simulink model "Hydraulic_Lift"  (R2013a)
settings: Solver=ode23t  StartTime=0.0  StopTime=20  MaxStep=0.02  RelTol=1e-3  AbsTol=1e-4
PreLoadFcn:
  | %cylinder_length = 15*2;
  | %piston_length = 15*2;
  | %leg_length = 15*2;
  | %platform_length = 25*2;
PostLoadFcn:
  | warning off sm:compiler:topologyAnalysis:DanglingBlock
  | warning off Simulink:SL_SolverMaskedZC;
  | warning off Simulink:SL_SolverIgnoredZCBracketing;
  | warning off Simulink:Engine:SolverMinStepNonlinearIterWarnForDAE;
  | warning off simscape:compiler:sli:init:SolverNotRecommended
  | warning off Simulink:Engine:UsingDiscreteSolver
  | load_system('Cylinder_Lib');
  | load_system('Motor_Lib');
  | load_system('Valve_Lib');
  | load_system('Load_Lib');
undefined symbols (not defined in the file or in its folder): Local, Scissor_Lift_Param, sigbuilder_block, X, Y, Z
libraries: fl_lib x80, sm_lib x41, Scissor_Parts_Lib x24, nesl_utility x8, Custom_lib x1
(part 1 of 2)
Description:
  | Copyright 2013 The MathWorks, Inc.
settings Model: Creator=smiller  LastModifiedBy=smiller
settings OptimizationCC: ExpressionDepthLimit=2147483647
settings SimscapeCC: SimscapeLogType=all  SimscapeLogSimulationStatistics=on  SimscapeLogLimitData=off
settings ExplorerConfigSet: InternalSimMechanicsExplorerSettings="<ExplorerConfiguration><canonicalview>default</canonicalview><TilePanel><TileInfo><Tiles Columns=\"1\" Count=\"1\" Rows=\"1\"><Column Left=\"2\" Weight=\"1\"/><Column Left=\"424\"/><Row Top=\"2\" Weight=\"1\"/><Row Top=\"524\"/><Tile Height=\"1\" Width=\"1\" X=\"0\" Y=\"0\"/></Tiles></TileInfo><SceneInfo><SceneViewer><BGColor><R>0.94901961088180542</R><G>0.94901961088180542</G><B>0.94901961088180542</B></BGColor><Camera><Position><X>2.491802304979692</X><Y>-4.0942122250600148</Y><Z>2.1539121347282051</Z></Position><Center><X>-0.87035068779914659</X><Y>-0.07952129192366976</Y><Z>1.2617431921759128</Z></Center><Up><X>-0.14501327569823058</X><Y>0.097366663542222315</Y><Z>0.98462728110789444</Z></Up><Left>-1.3650000751018525</Left><Right>1.3650000751018525</Right><Bottom>-1.2464621901512147</Bottom><Top>1.2464621901512147</Top></Camera></SceneViewer></SceneInfo></TilePanel></ExplorerConfiguration>"

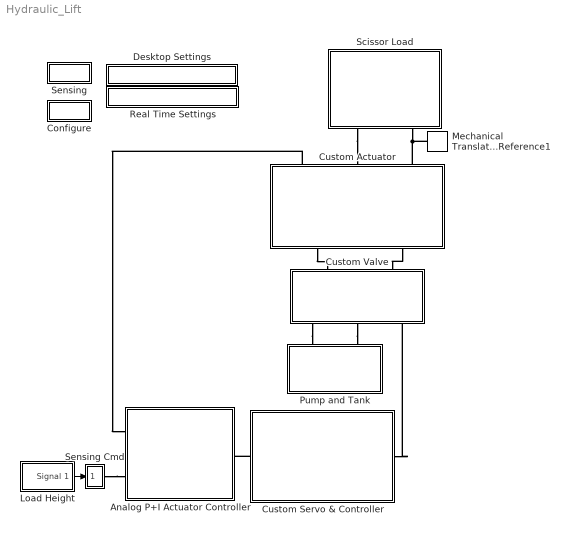
== system Hydraulic_Lift ==
  Analog P+I Actuator Controller : Subsystem
      mask Display: image(imread('Analog_PI_Controller_IMAGE.jpg'))
  Configure : Subsystem
      settings: OpenFcn=|
      | set_param([bdroot '/Configure/Commands'],'Location',[543 426 1032 720]);
      | open_system([bdroot '/Configure/Commands'],'window');
  Custom Actuator : Subsystem  mask(Double-Acting Hydraulic Actuator){A=5e-4, V=10e-6, PA=200, PB=0, T=200}
      mask prompts: A "Piston area (m^2)"; V "Chamber dead volume (m^3)"; PA "Positive-acting chamber A inital pressure (bar)"; PB "Negative-acting chamber B inital pressure (bar)"; T "Piston Travel (mm)"
      mask help: Models a double-acting hydraulic actuator using foundation libary blocks
      mask Display: image(imread('Double_Acting_Cylinder_Custom_IMAGE.jpg'));
  Custom Servo & Controller : Subsystem  mask{G=0.5e-3/(pi/2), J=1e-4, lambda=0.01, R=10, L=2.5, Kt=0.04, R_controller=[10e3 10e3 10e3 100e3 50 100e3 10e3], x_max=0.5}
      mask prompts: G "Spool displacement per motor rotation"; J "Total inertia reflected to motor (kg m^2)"; lambda "Total damping reflected to motor (Nm/(rad/s))"; R "Torque motor winding resistance (ohms)"; L "Torque motor winding inductance (H)"; Kt "Torque motor torque constant (Nm/A)"; R_controller "Motor controller resistance values [R1 R2 R3 R4 R5 R6 R7] (ohms)"; x_max "Spool displacement limit (mm)"
      mask Display: image(imread('DC_Motor_Custom_IMAGE.jpg'))
  Custom Valve : Subsystem  mask(Single-Stage Servo Valve){K_V=0.5, x_max=0.5, A_max=9, x_lap=0.02, A_leak=0.25}
      mask prompts: K_V "Flow Coefficient:"; x_max "Spool displacement limit (mm)"; A_max "Maximum oriface area (mm^2)"; x_lap "Spool displacement range for leakage (mm)"; A_leak "Leakage area at x=0 (mm^2)"
      mask help: Models a spool valve actuated directly by a torque motor.
      mask Display: image(imread('Four_Way_Valve_Custom_IMAGE.jpg'))
  Desktop Settings : Subsystem
      settings: OpenFcn=|
      | set_param(bdroot,'Solver','ODE23t','MaxStep','0.02');
      | 
      | 
      | tvar_solverBlock = find_system(bdroot, 'SubClassName', 'solver');
      | 
      | for i=1:size(tvar_solverBlock,1)
      | 
      | set_param(char(tvar_solverBlock(i)), 'UseLocalSolver','off','DoFixedCost','off');
      | end
      | 
      | clear tvar_solverBlock
      mask Display: disp('Desktop Settings')
  Load Height : Subsystem  Tag=STV Subsys  LoadFcn=sigbuilder_block('load');  StartFcn=sigbuilder_block('start');  StopFcn=sigbuilder_block('stop');  ClipboardFcn=sigbuilder_block('clipboard');  mask(Sigbuilder block){}
      mask help: Sigbuilder GUI
      mask init:
      | if ~strcmp(get_param(bdroot(gcbh),'SimulationStatus'),'stopped') tuvar = sigbuilder_block('maskInit'); end
      settings: CopyFcn=sigbuilder_block('copy');  DeleteFcn=sigbuilder_block('delete');  ModelCloseFcn=sigbuilder_block('modelClose');  PreSaveFcn=sigbuilder_block('preSave');  PauseFcn=sigbuilder_block('pause')  ContinueFcn=sigbuilder_block('continue')  NameChangeFcn=sigbuilder_block('namechange');  OpenFcn=sigbuilder_block('open',[181.241 5.58621 330.828 249.517 ]);  CloseFcn=sigbuilder_block('close');
      mask Display: plot(0,0,100,100,[10,10,40,40,10],[80,20,20,80,80],[40,10],[50,50], [40,27,10],[65,72,56],[40,25,25,10],[28,28,43,43]);
  Mechanical Translational Reference1 : fl_lib/Mechanical/Translational Elements/Mechanical Translational Reference  f_Log=off  LocalVarNames=|f  LocalVarDescs=|f  LocalVarLogging=[]
  Pump and Tank : Subsystem
      mask Display: image(imread('Pump_IMAGE.JPG'));
  Real Time Settings : Subsystem
      settings: OpenFcn=|
      | tvar_Nonlinear_Iterations = '4';
      | tvar_StepSize = '0.002';
      | %tvar_LocalSolver = 'NE_TRAPEZOIDAL_ADVANCER';
      | tvar_LocalSolver = 'NE_BACKWARD_EULER_ADVANCER';
      | 
      | set_param(bdroot,'Solver','ode1','FixedStep','auto');
      | 
      | tvar_solverBlock = find_system(bdroot, 'SubClassName', 'solver');
      | for i=1:size(tvar_solverBlock,1)
      | 
      | set_param(char(tvar_solverBlock(i)), 'UseLocalSolver','on','DoFixedCost','on','MaxNonlinIter',tvar_Nonlinear_Iterations,'LocalSolverChoice',tvar_LocalSolver,'LocalSolverSampleTime',tvar_StepSize);
      | end
      | clear tvar_Nonlinear_Iterations tvar_StepSize tvar_LocalSolver tvar_solverBlock
      mask Display: disp('Real Time Settings')
  Scissor Load : Subsystem
      mask Display: image(imread('Load_Scissor_IMAGE.JPG'));
  Sensing : Subsystem
  Sensing Cmd : Subsystem
      mask Display: disp('S')
  wires:
  Load Height/1(Signal 1) -> Sensing Cmd/1(In1)
  connections:
  Mechanical Translational Reference1/LConn1 -- Scissor Load/LConn2 -- Custom Actuator/RConn3
  Custom Actuator/LConn1 -- Custom Valve/RConn1
  Custom Servo & Controller/LConn1 -- Analog P+I Actuator Controller/RConn1
  Custom Actuator/LConn2 -- Custom Valve/RConn2
  Custom Actuator/RConn1 -- Analog P+I Actuator Controller/LConn1
  Sensing Cmd/RConn1 -- Analog P+I Actuator Controller/LConn2
  Scissor Load/LConn1 -- Custom Actuator/RConn2
  Custom Valve/LConn1 -- Pump and Tank/RConn1
  Custom Valve/LConn2 -- Pump and Tank/RConn2
  Custom Servo & Controller/RConn1 -- Custom Valve/LConn3

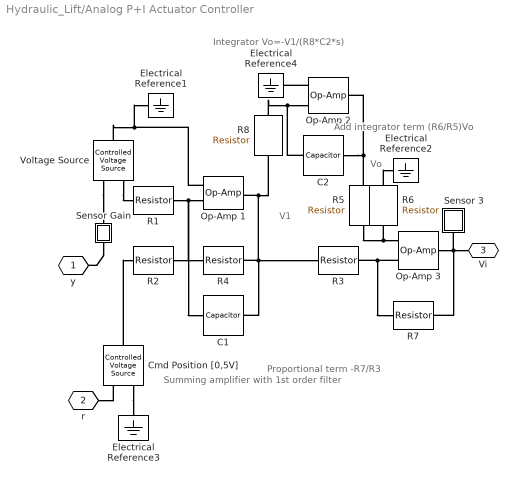
== system Hydraulic_Lift/Analog P+I Actuator Controller ==
  note: Summing amplifier
      | with 1st order filter
  note: Integrator
      | Vo=-V1/(R8*C2*s)
  note: Proportional
      | term -R7/R3
  note: Add integrator
      | term (R6/R5)Vo
  note: Vo
  note: V1
  C1 : fl_lib/Electrical/Electrical Elements/Capacitor  c=0.15e-06 F  v0=0 V  r=1e-06 Ohm  g=0 1/Ohm  i_Log=off  v_Log=off  vc_Log=off  LocalVarNames=|current|voltage|power  LocalVarDescs=|Capacitor current (A)|Voltage across capacitor (V)|Power (W)  LocalVarLogging=[0 0 0]
  C2 : fl_lib/Electrical/Electrical Elements/Capacitor  c=100e-06 F  v0=0 V  r=1e-06 Ohm  g=0 1/Ohm  i_Log=off  v_Log=off  vc_Log=off  LocalVarNames=|current|voltage|power  LocalVarDescs=|Capacitor current (A)|Voltage across capacitor (V)|Power (W)  LocalVarLogging=[0 0 0]
  Cmd Position [0,5V] : fl_lib/Electrical/Electrical Sources/Controlled Voltage Source  i_Log=off  v_Log=off  LocalVarNames=|current|voltage|power  LocalVarDescs=|Current (A)|Voltage (V)|Power (W)  LocalVarLogging=[0 0 0]
  Electrical Reference{1..4} (4 alike) : fl_lib/Electrical/Electrical Elements/Electrical Reference  i_Log=off  LocalVarNames=|i  LocalVarDescs=|i  LocalVarLogging=[]
  Op-Amp 1 : fl_lib/Electrical/Electrical Elements/Op-Amp  i1_Log=off  v1_Log=off  outI_Log=off  LocalVarNames=|i1|v1|outI  LocalVarDescs=|i1|v1|outI  LocalVarLogging=[]
  Op-Amp 2 : fl_lib/Electrical/Electrical Elements/Op-Amp  i1_Log=off  v1_Log=off  outI_Log=off  LocalVarNames=|i1|v1|outI  LocalVarDescs=|i1|v1|outI  LocalVarLogging=[]
  Op-Amp 3 : fl_lib/Electrical/Electrical Elements/Op-Amp  i1_Log=off  v1_Log=off  outI_Log=off  LocalVarNames=|i1|v1|outI  LocalVarDescs=|i1|v1|outI  LocalVarLogging=[]
  R{1..3,5..6,8} (6 alike) : fl_lib/Electrical/Electrical Elements/Resistor  R=10e3 Ohm  i_Log=off  v_Log=off  LocalVarNames=|current|voltage|power  LocalVarDescs=|Resistor current (A)|Voltage across resistor (V)|Power (W)  LocalVarLogging=[0 0 0]
  R4 : fl_lib/Electrical/Electrical Elements/Resistor  R=5.7e3 Ohm  i_Log=off  v_Log=off  LocalVarNames=|current|voltage|power  LocalVarDescs=|Resistor current (A)|Voltage across resistor (V)|Power (W)  LocalVarLogging=[0 0 0]
  R7 : fl_lib/Electrical/Electrical Elements/Resistor  R=20e3 Ohm  i_Log=off  v_Log=off  LocalVarNames=|current|voltage|power  LocalVarDescs=|Resistor current (A)|Voltage across resistor (V)|Power (W)  LocalVarLogging=[0 0 0]
  Sensor Gain : Subsystem
      mask Display: disp('G')
  Sensor 3 : Subsystem
      mask Display: disp('S')
  Voltage Source : fl_lib/Electrical/Electrical Sources/Controlled Voltage Source  i_Log=off  v_Log=off  LocalVarNames=|current|voltage|power  LocalVarDescs=|Current (A)|Voltage (V)|Power (W)  LocalVarLogging=[0 0 0]
  y : PMIOPort  Tag=PMCPort  Port=1  Side=Left
  r : PMIOPort  Tag=PMCPort  Port=2  Side=Left
  Vi : PMIOPort  Port=3  Side=Right
  connections:
  r/RConn1 -- Cmd Position [0,5V]/RConn1
  Vi/RConn1 -- R7/RConn1 -- Op-Amp 3/RConn1 -- Sensor 3/LConn1
  R1/RConn1 -- R2/RConn1 -- R4/LConn1 -- C1/LConn1 -- Op-Amp 1/LConn2
  R4/RConn1 -- R3/LConn1 -- C1/RConn1 -- R8/LConn1 -- Op-Amp 1/RConn1
  R8/RConn1 -- C2/LConn1 -- Op-Amp 2/LConn2
  C2/RConn1 -- R5/LConn1 -- Op-Amp 2/RConn1
  Op-Amp 1/LConn1 -- Voltage Source/LConn1 -- Electrical Reference1/LConn1
  R5/RConn1 -- R6/LConn1 -- Op-Amp 3/LConn1
  Op-Amp 3/LConn2 -- R7/LConn1 -- R3/RConn1
  Voltage Source/RConn2 -- R1/LConn1
  Cmd Position [0,5V]/LConn1 -- R2/LConn1
  Cmd Position [0,5V]/RConn2 -- Electrical Reference3/LConn1
  R6/RConn1 -- Electrical Reference2/LConn1
  Op-Amp 2/LConn1 -- Electrical Reference4/LConn1
  Voltage Source/RConn1 -- Sensor Gain/RConn1
  Sensor Gain/LConn1 -- y/RConn1

== system Hydraulic_Lift/Configure ==
  Commands : Subsystem

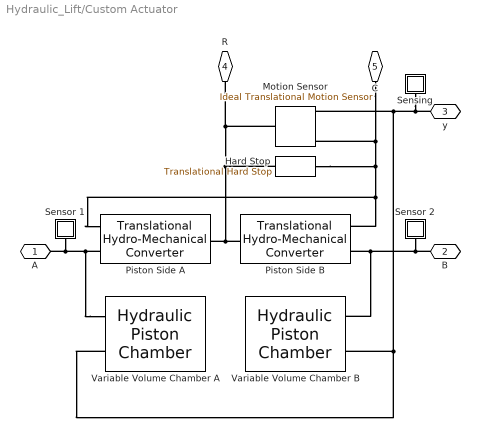
== system Hydraulic_Lift/Custom Actuator ==
  " Motion Sensor" : fl_lib/Mechanical/Mechanical Sensors/Ideal Translational Motion Sensor  offset=Scissor_Lift_Param.Initial_Cyl_Ext mm  v_Log=off  f_Log=off  x_Log=off  LocalVarNames=|v|f|x  LocalVarDescs=|v|f|x  LocalVarLogging=[]
  Hard Stop : fl_lib/Mechanical/Translational Elements/Translational Hard Stop  upper_bnd=T/2 mm  lower_bnd=-T/2 mm  stiff_up=1e7 N/m  stiff_low=1e7 N/m  D_up=1500 N/(m/s)  D_low=1500 N/(m/s)  initial_position=0 m  f_Log=off  v_Log=off  x_Log=off  LocalVarNames=|f|v|x  LocalVarDescs=|f|v|x  LocalVarLogging=[0 0 0]
  Piston Side A : fl_lib/Hydraulic/Hydraulic Elements/Translational Hydro-Mechanical Converter  area=A m^2  or=1  dir=1  f_Log=off  q_Log=off  LocalVarNames=|flow_rate|pressure|force|power  LocalVarDescs=|Flow rate into the chamber (m^3/s)|Pressure at the inlet (Pa)|Output force (N)|Power (W)  LocalVarLogging=[0 0 0 0]
  Piston Side B : fl_lib/Hydraulic/Hydraulic Elements/Translational Hydro-Mechanical Converter  area=A m^2  or=2  dir=1  f_Log=off  q_Log=off  LocalVarNames=|flow_rate|pressure|force|power  LocalVarDescs=|Flow rate into the chamber (m^3/s)|Pressure at the inlet (Pa)|Output force (N)|Power (W)  LocalVarLogging=[0 0 0 0]
  Sensing : Subsystem
      mask Display: disp('S')
  Sensor 1 : Subsystem
      mask Display: disp('S')
  Sensor 2 : Subsystem
      mask Display: disp('S')
  Variable Volume Chamber A : fl_lib/Hydraulic/Hydraulic Elements/Hydraulic Piston Chamber  area=A m^2  init_pos=0 m  or=1  V_dead=V m^3  k_sh=1.4  initial_pressure=PA bar  x_or=1  p_a=101325.0 Pa  chamber_flow_rate_Log=off  pressure_chamber_Log=off  LocalVarNames=|flow_rate|pressure|volume|fl_volume  LocalVarDescs=|Flow rate into the chamber (m^3/s)|Pressure at the inlet (Pa)|Instantaneous chamber volume (m^3)|Compressed fluid volume (m^3)  LocalVarLogging=[0 0 0 0]
  Variable Volume Chamber B : fl_lib/Hydraulic/Hydraulic Elements/Hydraulic Piston Chamber  area=A m^2  init_pos=0 m  or=2  V_dead=V m^3  k_sh=1.4  initial_pressure=PB bar  x_or=1  p_a=101325.0 Pa  chamber_flow_rate_Log=off  pressure_chamber_Log=off  LocalVarNames=|flow_rate|pressure|volume|fl_volume  LocalVarDescs=|Flow rate into the chamber (m^3/s)|Pressure at the inlet (Pa)|Instantaneous chamber volume (m^3)|Compressed fluid volume (m^3)  LocalVarLogging=[0 0 0 0]
  A : PMIOPort  Port=1  Side=Left
  B : PMIOPort  Port=2  Side=Left
  y : PMIOPort  Port=3  Side=Right
  R : PMIOPort  Port=4  Side=Right
  C : PMIOPort  Port=5  Side=Right
  connections:
  Variable Volume Chamber A/LConn1 -- Sensing/LConn1 -- y/RConn1 -- " Motion Sensor"/RConn3 -- Variable Volume Chamber B/LConn1
  " Motion Sensor"/LConn1 -- R/RConn1 -- Piston Side A/RConn1 -- Piston Side B/RConn1 -- Hard Stop/LConn1
  Piston Side A/LConn1 -- Hard Stop/RConn1 -- C/RConn1 -- " Motion Sensor"/RConn1 -- Piston Side B/LConn1
  Variable Volume Chamber B/LConn2 -- Sensor 2/LConn1 -- B/RConn1 -- Piston Side B/LConn2
  Variable Volume Chamber A/LConn2 -- Piston Side A/LConn2 -- A/RConn1 -- Sensor 1/LConn1

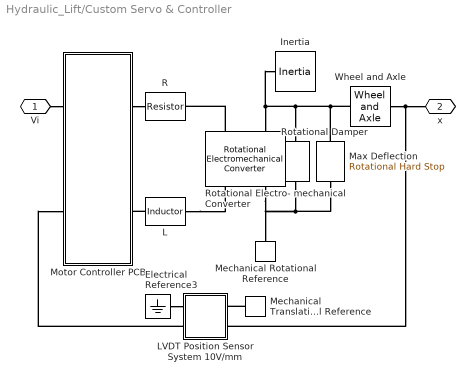
== system Hydraulic_Lift/Custom Servo & Controller ==
  Electrical Reference3 : fl_lib/Electrical/Electrical Elements/Electrical Reference  i_Log=off  LocalVarNames=|i  LocalVarDescs=|i  LocalVarLogging=[]
  Inertia : fl_lib/Mechanical/Rotational Elements/Inertia  inertia=J kg*m^2  initial_velocity=0 rad/s  t_Log=off  LocalVarNames=|torque|velocity  LocalVarDescs=|Inertia torque (N*m)|Inertia absolute velocity (rad/s)  LocalVarLogging=[0 0]
  L : fl_lib/Electrical/Electrical Elements/Inductor  l=L H  i0=0 A  r=0 Ohm  g=1e-09 1/Ohm  i_Log=off  v_Log=off  i_L_Log=off  LocalVarNames=|current|voltage|power  LocalVarDescs=|Inductor current (A) |Voltage across inductor (V)|Power (W)  LocalVarLogging=[0 0 0]
  LVDT Position Sensor System 10V/mm : Subsystem
  Max Deflection : fl_lib/Mechanical/Rotational Elements/Rotational Hard Stop  upper_bnd=x_max*1e-3/G rad  lower_bnd=-x_max*1e-3/G rad  stiff_up=1e+06 N*m/rad  stiff_low=1e+06 N*m/rad  D_up=0.05 N*m/(rad/s)  D_low=0.05 N*m/(rad/s)  initial_angle=0 rad  t_Log=off  w_Log=off  phi_Log=off  LocalVarNames=|contact_torque|rel_angle  LocalVarDescs=|Contact torque (N*m)|Slider-case relative angle (rad)  LocalVarLogging=[0 0]
  Mechanical Rotational Reference : fl_lib/Mechanical/Rotational Elements/Mechanical Rotational Reference  t_Log=off  LocalVarNames=|t  LocalVarDescs=|t  LocalVarLogging=[]
  Mechanical Translational Reference : fl_lib/Mechanical/Translational Elements/Mechanical Translational Reference  f_Log=off  LocalVarNames=|f  LocalVarDescs=|f  LocalVarLogging=0
  Motor Controller PCB : Subsystem
  R : fl_lib/Electrical/Electrical Elements/Resistor  Tag=Factory Generic  R=R Ohm  i_Log=off  v_Log=off  LocalVarNames=|current|voltage|power  LocalVarDescs=|Resistor current (A)|Voltage across resistor (V)|Power (W)  LocalVarLogging=[0 0 0]
  Rotational Damper : fl_lib/Mechanical/Rotational Elements/Rotational Damper  D=lambda N*m/(rad/s)  t_Log=off  w_Log=off  LocalVarNames=|torque|velocity|power  LocalVarDescs=|Damping torque (N*m)|Damper relative velocity (rad/s)|Power dissipated in the damper (W)  LocalVarLogging=[0 0 0]
  Rotational Electro- mechanical Converter : fl_lib/Electrical/Electrical Elements/Rotational Electromechanical Converter  K=Kt V/(rad/s)  i_Log=off  v_Log=off  t_Log=off  w_Log=off  LocalVarNames=|current|voltage|power|torque|speed  LocalVarDescs=|Current (A)|Voltage (V)|Power (W)|Torque (Nm)|Angular speed (rad/s)  LocalVarLogging=[0 0 0 0 0]
  Wheel and Axle : fl_lib/Mechanical/Mechanisms/Wheel and Axle  R=G m  or=1  orient=1  t_Log=off  f_Log=off  LocalVarNames=|t|f  LocalVarDescs=|t|f  LocalVarLogging=[0 0]
  Vi : PMIOPort  Port=1  Side=Left
  x : PMIOPort  Port=2  Side=Right
  connections:
  LVDT Position Sensor System 10V/mm/RConn2 -- Motor Controller PCB/LConn2
  Electrical Reference3/LConn1 -- LVDT Position Sensor System 10V/mm/RConn1
  Vi/RConn1 -- Motor Controller PCB/LConn1
  Motor Controller PCB/RConn1 -- R/LConn1
  Rotational Electro- mechanical Converter/LConn1 -- R/RConn1
  Max Deflection/RConn1 -- Rotational Damper/RConn1 -- Rotational Electro- mechanical Converter/RConn2 -- Mechanical Rotational Reference/LConn1
  Max Deflection/LConn1 -- Inertia/LConn1 -- Rotational Electro- mechanical Converter/LConn2 -- Rotational Damper/LConn1 -- Wheel and Axle/LConn1
  L/LConn1 -- Motor Controller PCB/RConn2
  L/RConn1 -- Rotational Electro- mechanical Converter/RConn1
  Wheel and Axle/RConn1 -- LVDT Position Sensor System 10V/mm/LConn2 -- x/RConn1
  Mechanical Translational Reference/LConn1 -- LVDT Position Sensor System 10V/mm/LConn1

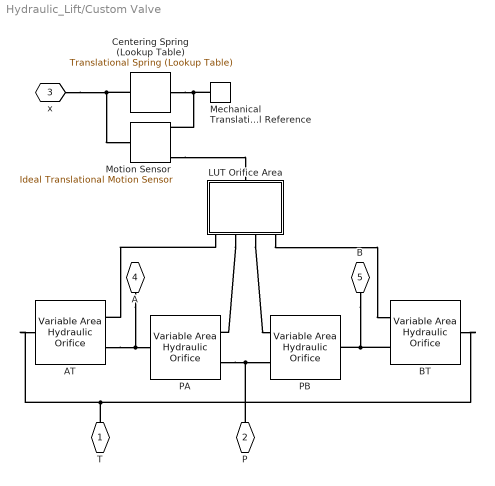
== system Hydraulic_Lift/Custom Valve ==
  AT : fl_lib/Hydraulic/Hydraulic Elements/Variable Area Hydraulic Orifice  C_d=K_V  Re_cr=12  C_d_lam=0.0408  min_area=1e-12 m^2  q_Log=off  p_Log=off  LocalVarNames=|flow_rate|pr_drop|power  LocalVarDescs=|Flow rate through the orifice (m^3)|Pressure drop across the orifice (Pa)|Power dissipated in the orifice (W)  LocalVarLogging=[0 0 0]
  BT : fl_lib/Hydraulic/Hydraulic Elements/Variable Area Hydraulic Orifice  C_d=K_V  Re_cr=12  C_d_lam=0.0408  min_area=1e-12 m^2  q_Log=off  p_Log=off  LocalVarNames=|flow_rate|pr_drop|power  LocalVarDescs=|Flow rate through the orifice (m^3)|Pressure drop across the orifice (Pa)|Power dissipated in the orifice (W)  LocalVarLogging=[0 0 0]
  Centering Spring (Lookup Table) : Custom_lib/Mechanical/Translational Spring (Lookup Table)  xd=[-1 -0.9 0,0.9 1]*x_max mm  kd=[100,10,10,10,100] N/m  x0=0 m  f_Log=off  x_Log=off  v_Log=off  k_Log=off  LocalVarNames=|f|x|v|k  LocalVarDescs=|Force through variable|Displacement|Velocity across variable|Spring Stiffness  LocalVarLogging=[0 0 0 0]
  LUT Orifice Area : Subsystem
  Mechanical Translational Reference : fl_lib/Mechanical/Translational Elements/Mechanical Translational Reference  f_Log=off  LocalVarNames=|f  LocalVarDescs=|f  LocalVarLogging=0
  Motion Sensor : fl_lib/Mechanical/Mechanical Sensors/Ideal Translational Motion Sensor  offset=0 m  v_Log=off  f_Log=off  x_Log=off  LocalVarNames=|v|f|x  LocalVarDescs=|v|f|x  LocalVarLogging=[0 0 0]
  PA : fl_lib/Hydraulic/Hydraulic Elements/Variable Area Hydraulic Orifice  C_d=K_V  Re_cr=12  C_d_lam=0.0408  min_area=1e-12 m^2  q_Log=off  p_Log=off  LocalVarNames=|flow_rate|pr_drop|power  LocalVarDescs=|Flow rate through the orifice (m^3)|Pressure drop across the orifice (Pa)|Power dissipated in the orifice (W)  LocalVarLogging=[0 0 0]
  PB : fl_lib/Hydraulic/Hydraulic Elements/Variable Area Hydraulic Orifice  C_d=K_V  Re_cr=12  C_d_lam=0.0408  min_area=1e-12 m^2  q_Log=off  p_Log=off  LocalVarNames=|flow_rate|pr_drop|power  LocalVarDescs=|Flow rate through the orifice (m^3)|Pressure drop across the orifice (Pa)|Power dissipated in the orifice (W)  LocalVarLogging=[0 0 0]
  T : PMIOPort  Tag=PMCPort  Port=1  Side=Left
  P : PMIOPort  Tag=PMCPort  Port=2  Side=Left
  x : PMIOPort  Tag=PMCPort  Port=3  Side=Left
  A : PMIOPort  Tag=PMCPort  Port=4  Side=Right
  B : PMIOPort  Tag=PMCPort  Port=5  Side=Right
  connections:
  AT/RConn1 -- BT/RConn1 -- T/RConn1
  AT/LConn2 -- PA/RConn1 -- A/RConn1
  PA/LConn2 -- P/RConn1 -- PB/LConn2
  B/RConn1 -- BT/LConn2 -- PB/RConn1
  Mechanical Translational Reference/LConn1 -- Centering Spring (Lookup Table)/RConn1 -- Motion Sensor/RConn1
  LUT Orifice Area/RConn1 -- AT/LConn1
  LUT Orifice Area/RConn4 -- BT/LConn1
  LUT Orifice Area/RConn2 -- PA/LConn1
  LUT Orifice Area/RConn3 -- PB/LConn1
  x/RConn1 -- Centering Spring (Lookup Table)/LConn1 -- Motion Sensor/LConn1
  Motion Sensor/RConn3 -- LUT Orifice Area/LConn1

== system Hydraulic_Lift/Desktop Settings ==

== system Hydraulic_Lift/Load Height ==
  Demux : Demux  Tag=STV Demux  Outputs=1
  FromWs : FromWorkspace  Tag=STV FromWs  VariableName=tuvar  SampleTime=0
      SigBuilderData=|
      | common.afterFinalStr = 'Extrapolate'
      | common.sampleTime = 0
      | dataSet.timeRange = [0 20]
      | dataSet.name = 'Group 1'
      | sbobj.Groups.Name = 'Group 1'
      | sbobj.Groups.Signals.Name = 'Signal 1'
      | sbobj.Groups.Signals.XData = [0 1 3 4 10 12 15 20]
      | sbobj.Groups.Signals.YData = [2.5 2.5 5 5 0 0 2.5 2.5]
      | sbobj.Groups.TimeRange = [0 20]
  Signal 1 : Outport  Tag=STV Outport
  wires:
  Demux/1 -> Signal 1/1
  FromWs/1 -> Demux/1

== system Hydraulic_Lift/Pump and Tank ==
  Custom Hydraulic Fluid : fl_lib/Hydraulic/Hydraulic Utilities/Custom Hydraulic Fluid  density=850 kg/m^3  viscosity_kin=1.8e-05 m^2/s  bulk=8e+08 Pa  alpha=0.005  LocalVarLogging=[]
  Hydraulic Reference : fl_lib/Hydraulic/Hydraulic Elements/Hydraulic Reference  q_Log=off  LocalVarNames=|q  LocalVarDescs=|q  LocalVarLogging=[]
  Pump : fl_lib/Hydraulic/Hydraulic Sources/Hydraulic Pressure Source  q_Log=off  p_Log=off  LocalVarNames=|flow_rate|pr_differential|power  LocalVarDescs=|Flow rate through the source (m^3/s)|Pressure differential across the source (Pa)|Source power (W)  LocalVarLogging=[0 0 0]
  Solver Configuration : nesl_utility/Solver Configuration  PhysicalDomain=network_engine_domain  SubClassName=solver  LeftPortType=input  RightPortType=generic  Accelerate=off  Tones=[]  Harmonics=[]  SimulateNoise=off  Profile=off  UseLocalSampling=off  EnableSwitchedLinearOptims=on  FrequencyDomain=off  UseCCode=off  UseNewInitialization=off  DoDC=off  ResidualTolerance=1e-9  UseLocalSolver=off  LocalSolverChoice=NE_BACKWARD_EULER_ADVANCER  LocalSolverSampleTime=0.002  DoFixedCost=off  MaxNonlinIter=4  MaxModeIter=2  LinearAlgebra=Sparse  DelaysMemoryBudget=1024
  Supply Pressure : Constant  Value=200
  bar : nesl_utility/Simulink-PS Converter  PhysicalDomain=network_engine_domain  SubClassName=ps_input  LeftPortType=input  RightPortType=output  PseudoPeriodic=off  Frequencies=[]  NoiseDistribution=none  NoiseParameters=[]  Unit=bar  AffineConversion=off  InputFiltering=off  SimscapeFilterOrder=1  InputFilterTimeConstant=.001  UdotUserProvided=0
  T : PMIOPort  Port=1  Side=Right
  P : PMIOPort  Port=2  Side=Right
  wires:
  Supply Pressure/1 -> bar/1
  connections:
  bar/RConn1 -- Pump/RConn1
  Pump/RConn2 -- T/RConn1 -- Custom Hydraulic Fluid/RConn1 -- Solver Configuration/RConn1 -- Hydraulic Reference/LConn1
  Pump/LConn1 -- P/RConn1

== system Hydraulic_Lift/Real Time Settings ==

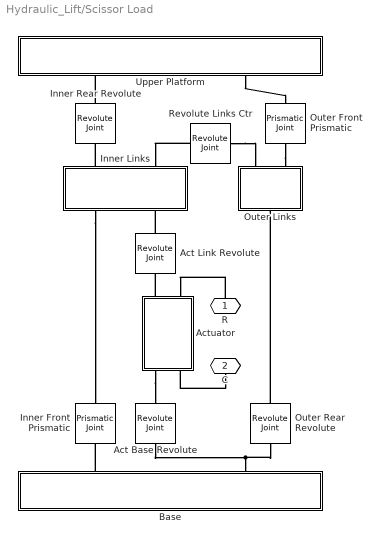
== system Hydraulic_Lift/Scissor Load ==
  Act Base Revolute : sm_lib/Joints/Revolute Joint  SenseConstraintForceX=off  SenseConstraintForceY=off  SenseConstraintForceZ=off  SenseConstraintTorqueX=off  SenseConstraintTorqueY=off  SenseConstraintTorqueZ=off  ConstraintWrenchDir=FollowerOnBase  ConstraintWrenchFrame=BaseFrame  EquilibriumPosition=0  EquilibriumPositionUnits=deg  SpringStiffness=0  SpringStiffnessUnits=N*m/deg  DampingCoefficient=0  DampingCoefficientUnits=N*m/(deg/s)  ActuationMode=NoActuation  SensePosition=off  SenseVelocity=off  SenseAcceleration=off  SenseTorqueForce=off  PositionTargetValue=0  PositionTargetValueUnits=deg  PositionTargetSpecify=off  PositionTargetPriority=High  VelocityTargetValue=0  VelocityTargetValueUnits=deg/s  VelocityTargetSpecify=off  VelocityTargetPriority=High  BlockFunction=simmechanics.library.joints.revolute_joint
  Act Link Revolute : sm_lib/Joints/Revolute Joint  SenseConstraintForceX=off  SenseConstraintForceY=off  SenseConstraintForceZ=off  SenseConstraintTorqueX=off  SenseConstraintTorqueY=off  SenseConstraintTorqueZ=off  ConstraintWrenchDir=FollowerOnBase  ConstraintWrenchFrame=BaseFrame  EquilibriumPosition=0  EquilibriumPositionUnits=deg  SpringStiffness=0  SpringStiffnessUnits=N*m/deg  DampingCoefficient=0  DampingCoefficientUnits=N*m/(deg/s)  ActuationMode=NoActuation  SensePosition=off  SenseVelocity=off  SenseAcceleration=off  SenseTorqueForce=off  PositionTargetValue=0  PositionTargetValueUnits=deg  PositionTargetSpecify=off  PositionTargetPriority=High  VelocityTargetValue=0  VelocityTargetValueUnits=deg/s  VelocityTargetSpecify=off  VelocityTargetPriority=High  BlockFunction=simmechanics.library.joints.revolute_joint
  Actuator : Subsystem
  Base : Subsystem
  Inner Links : Subsystem
  "Inner Front Prismatic " : sm_lib/Joints/Prismatic  Joint  SenseConstraintForceX=off  SenseConstraintForceY=off  SenseConstraintForceZ=off  SenseConstraintTorqueX=off  SenseConstraintTorqueY=off  SenseConstraintTorqueZ=off  ConstraintWrenchDir=FollowerOnBase  ConstraintWrenchFrame=BaseFrame  EquilibriumPosition=0  EquilibriumPositionUnits=m  SpringStiffness=0  SpringStiffnessUnits=N/m  DampingCoefficient=0  DampingCoefficientUnits=N/(m/s)  ActuationMode=NoActuation  SensePosition=off  SenseVelocity=off  SenseAcceleration=off  SenseTorqueForce=off  PositionTargetValue=0  PositionTargetValueUnits=m  PositionTargetSpecify=off  PositionTargetPriority=High  VelocityTargetValue=0  VelocityTargetValueUnits=m/s  VelocityTargetSpecify=off  VelocityTargetPriority=High  BlockFunction=simmechanics.library.joints.prismatic_joint
  Inner Rear Revolute : sm_lib/Joints/Revolute Joint  SenseConstraintForceX=off  SenseConstraintForceY=off  SenseConstraintForceZ=off  SenseConstraintTorqueX=off  SenseConstraintTorqueY=off  SenseConstraintTorqueZ=off  ConstraintWrenchDir=FollowerOnBase  ConstraintWrenchFrame=BaseFrame  EquilibriumPosition=0  EquilibriumPositionUnits=deg  SpringStiffness=0  SpringStiffnessUnits=N*m/deg  DampingCoefficient=0  DampingCoefficientUnits=N*m/(deg/s)  ActuationMode=NoActuation  SensePosition=off  SenseVelocity=off  SenseAcceleration=off  SenseTorqueForce=off  PositionTargetValue=15  PositionTargetValueUnits=deg  PositionTargetSpecify=off  PositionTargetPriority=Low  VelocityTargetValue=0  VelocityTargetValueUnits=deg/s  VelocityTargetSpecify=off  VelocityTargetPriority=High  BlockFunction=simmechanics.library.joints.revolute_joint
  Outer Links : Subsystem
  "Outer Front Prismatic " : sm_lib/Joints/Prismatic  Joint  SenseConstraintForceX=off  SenseConstraintForceY=off  SenseConstraintForceZ=off  SenseConstraintTorqueX=off  SenseConstraintTorqueY=off  SenseConstraintTorqueZ=off  ConstraintWrenchDir=FollowerOnBase  ConstraintWrenchFrame=BaseFrame  EquilibriumPosition=0  EquilibriumPositionUnits=m  SpringStiffness=0  SpringStiffnessUnits=N/m  DampingCoefficient=0  DampingCoefficientUnits=N/(m/s)  ActuationMode=NoActuation  SensePosition=off  SenseVelocity=off  SenseAcceleration=off  SenseTorqueForce=off  PositionTargetValue=0  PositionTargetValueUnits=m  PositionTargetSpecify=off  PositionTargetPriority=High  VelocityTargetValue=0  VelocityTargetValueUnits=m/s  VelocityTargetSpecify=off  VelocityTargetPriority=High  BlockFunction=simmechanics.library.joints.prismatic_joint
  Outer Rear Revolute : sm_lib/Joints/Revolute Joint  SenseConstraintForceX=off  SenseConstraintForceY=off  SenseConstraintForceZ=off  SenseConstraintTorqueX=off  SenseConstraintTorqueY=off  SenseConstraintTorqueZ=off  ConstraintWrenchDir=FollowerOnBase  ConstraintWrenchFrame=BaseFrame  EquilibriumPosition=0  EquilibriumPositionUnits=deg  SpringStiffness=0  SpringStiffnessUnits=N*m/deg  DampingCoefficient=0  DampingCoefficientUnits=N*m/(deg/s)  ActuationMode=NoActuation  SensePosition=off  SenseVelocity=off  SenseAcceleration=off  SenseTorqueForce=off  PositionTargetValue=-15  PositionTargetValueUnits=deg  PositionTargetSpecify=off  PositionTargetPriority=Low  VelocityTargetValue=0  VelocityTargetValueUnits=deg/s  VelocityTargetSpecify=off  VelocityTargetPriority=High  BlockFunction=simmechanics.library.joints.revolute_joint
  Revolute Links Ctr : sm_lib/Joints/Revolute Joint  SenseConstraintForceX=off  SenseConstraintForceY=off  SenseConstraintForceZ=off  SenseConstraintTorqueX=off  SenseConstraintTorqueY=off  SenseConstraintTorqueZ=off  ConstraintWrenchDir=FollowerOnBase  ConstraintWrenchFrame=BaseFrame  EquilibriumPosition=0  EquilibriumPositionUnits=deg  SpringStiffness=0  SpringStiffnessUnits=N*m/deg  DampingCoefficient=0  DampingCoefficientUnits=N*m/(deg/s)  ActuationMode=NoActuation  SensePosition=off  SenseVelocity=off  SenseAcceleration=off  SenseTorqueForce=off  PositionTargetValue=-2*Scissor_Lift_Param.Initial_Angle  PositionTargetValueUnits=deg  PositionTargetSpecify=on  PositionTargetPriority=Low  VelocityTargetValue=0  VelocityTargetValueUnits=deg/s  VelocityTargetSpecify=off  VelocityTargetPriority=High  BlockFunction=simmechanics.library.joints.revolute_joint
  Upper Platform : Subsystem
  R : PMIOPort  Port=1  Side=Left
  C : PMIOPort  Port=2  Side=Left
  connections:
  Act Base Revolute/LConn1 -- Base/RConn2 -- Outer Rear Revolute/LConn1
  Inner Links/RConn1 -- "Inner Front Prismatic "/LConn1
  Base/RConn1 -- "Inner Front Prismatic "/RConn1
  Upper Platform/LConn2 -- "Outer Front Prismatic "/RConn1
  "Outer Front Prismatic "/LConn1 -- Outer Links/RConn2
  Inner Rear Revolute/LConn1 -- Upper Platform/LConn1
  Inner Links/LConn1 -- Inner Rear Revolute/RConn1
  Outer Rear Revolute/RConn1 -- Outer Links/LConn1
  Revolute Links Ctr/RConn1 -- Outer Links/RConn1
  Revolute Links Ctr/LConn1 -- Inner Links/LConn2
  Actuator/RConn1 -- Act Link Revolute/RConn1
  Act Link Revolute/LConn1 -- Inner Links/RConn2
  Actuator/LConn1 -- Act Base Revolute/RConn1
  C/RConn1 -- Actuator/LConn2
  R/RConn1 -- Actuator/RConn2

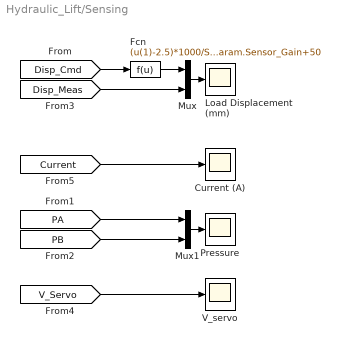
== system Hydraulic_Lift/Sensing ==
  Current (A) : Scope
      settings: YMin=-0.1  YMax=0.1
  Fcn : Fcn  Expr=(u(1)-2.5)*1000/Scissor_Lift_Param.Sensor_Gain+50
  Load Displacement (mm) : Scope
      settings: YMin=-100  YMax=200  SaveName=Hydraulic_Acutator_Analog_Control_DATA1
  Mux : Mux  Inputs=2
  Mux1 : Mux  Inputs=2
  Pressure : Scope
      settings: TimeRange=20  YMin=-50  YMax=250  SaveName=Hydraulic_Acutator_Analog_Control_DATA2
  V_servo : Scope
      settings: TimeRange=10  YMin=-0.2  YMax=0.2
  wires:
  [Disp_Meas] -> Mux/2
  Mux/1 -> Load Displacement (mm)/1
  Fcn/1 -> Mux/1
  [Disp_Cmd] -> Fcn/1
  Mux1/1 -> Pressure/1
  [PA] -> Mux1/1
  [PB] -> Mux1/2
  [V_Servo] -> V_servo/1
  [Current] -> Current (A)/1

== system Hydraulic_Lift/Sensing Cmd ==
  In1 : Inport
  Simulink-PS Converter : nesl_utility/Simulink-PS Converter  PhysicalDomain=network_engine_domain  SubClassName=ps_input  LeftPortType=input  RightPortType=output  PseudoPeriodic=off  Frequencies=[]  NoiseDistribution=none  NoiseParameters=[]  Unit=V  AffineConversion=off  InputFiltering=off  SimscapeFilterOrder=1  InputFilterTimeConstant=.001  UdotUserProvided=0
  Conn1 : PMIOPort  Port=1  Side=Right
  tag scope: Disp_Cmd=global
  wires:
  In1/1 -> [Disp_Cmd], Simulink-PS Converter/1
  connections:
  Simulink-PS Converter/RConn1 -- Conn1/RConn1

== system Hydraulic_Lift/Analog P+I Actuator Controller/Sensor Gain ==
  Initial Disp (m) : fl_lib/Physical Signals/Sources/PS Constant  constant=Scissor_Lift_Param.Initial_Cyl_Ext*1e-3  LocalVarLogging=[]
  Mid Range 2.5V : fl_lib/Physical Signals/Sources/PS Constant  constant=2.5  LocalVarLogging=[]
  PS Add : fl_lib/Physical Signals/Functions/PS Add  LocalVarLogging=[]
  PS Subtract : fl_lib/Physical Signals/Functions/PS Subtract  LocalVarLogging=[]
  Sensor Gain : fl_lib/Physical Signals/Functions/PS Gain  gain=Scissor_Lift_Param.Sensor_Gain  LocalVarLogging=[]
  Vout : PMIOPort  Port=1  Side=Right
  Din : PMIOPort  Port=2  Side=Left
  connections:
  PS Subtract/LConn1 -- Din/RConn1
  PS Subtract/RConn1 -- Sensor Gain/LConn1
  Vout/RConn1 -- PS Add/RConn1
  Initial Disp (m)/RConn1 -- PS Subtract/LConn2
  PS Add/LConn1 -- Sensor Gain/RConn1
  Mid Range 2.5V/RConn1 -- PS Add/LConn2

== system Hydraulic_Lift/Analog P+I Actuator Controller/Sensor 3 ==
  Electrical Reference3 : fl_lib/Electrical/Electrical Elements/Electrical Reference  i_Log=off  LocalVarNames=|i  LocalVarDescs=|i  LocalVarLogging=[]
  PS-Simulink Converter : nesl_utility/PS-Simulink Converter  PhysicalDomain=network_engine_domain  SubClassName=ps_output  LeftPortType=input  RightPortType=output  PseudoPeriodic=off  Frequencies=[]  Unit=1  AffineConversion=off
  Voltage Sensor : fl_lib/Electrical/Electrical Sensors/Voltage Sensor  i1_Log=off  v1_Log=off  LocalVarNames=|i1|v1  LocalVarDescs=|i1|v1  LocalVarLogging=[]
  + : PMIOPort  Port=1  Side=Left
  tag scope: V_Servo=global
  wires:
  PS-Simulink Converter/1 -> [V_Servo]
  connections:
  Voltage Sensor/RConn1 -- PS-Simulink Converter/LConn1
  +/RConn1 -- Voltage Sensor/LConn1
  Voltage Sensor/RConn2 -- Electrical Reference3/LConn1

== system Hydraulic_Lift/Configure/Commands ==
  note: Actuator
  note: Valve
  note: Motor
  note: Load
  Use Custom Actuator : Subsystem
      settings: OpenFcn=|
      | load_system('Cylinder_Lib');
      | load_system('Motor_Lib');
      | load_system('Valve_Lib');
      | load_system('Load_Lib');
      | 
      | bpth = replace_block(bdroot,'Name',sprintf('%s\n%s','Standard','Actuator'),'Cylinder_Lib/Custom','noprompt');
      | if(~isempty(bpth))
      | set_param(char(bpth),'Name',sprintf('%s\n%s','Custom','Actuator'),'LinkStatus','none');
      | end
      mask Display: disp('Custom')
  Use Custom Motor : Subsystem
      settings: OpenFcn=|
      | load_system('Cylinder_Lib');
      | load_system('Motor_Lib');
      | load_system('Valve_Lib');
      | load_system('Load_Lib');
      | 
      | bpth = replace_block(bdroot,'Name',sprintf('%s\n%s','Standard','Servo & Controller'),'Motor_Lib/Custom','noprompt');
      | if(~isempty(bpth))
      | set_param(char(bpth),'Name',sprintf('%s\n%s','Custom','Servo & Controller'),'LinkStatus','none');
      | end
      mask Display: disp('Custom')
  Use Custom Valve : Subsystem
      settings: OpenFcn=|
      | load_system('Cylinder_Lib');
      | load_system('Motor_Lib');
      | load_system('Valve_Lib');
      | load_system('Load_Lib');
      | 
      | bpth = replace_block(bdroot,'Name',sprintf('%s\n%s','Standard','Valve'),'Valve_Lib/Custom','noprompt');
      | if(~isempty(bpth))
      | set_param(char(bpth),'Name',sprintf('%s\n%s','Custom','Valve'),'LinkStatus','none');
      | end
      mask Display: disp('Custom')
  Use Scissor Load : Subsystem
      settings: OpenFcn=|
      | load_system('Cylinder_Lib');
      | load_system('Motor_Lib');
      | load_system('Valve_Lib');
      | load_system('Load_Lib');
      | 
      | bpth = replace_block(bdroot,'Name',sprintf('%s\n%s','Simple','Load'),'Load_Lib/Scissor','noprompt');
      | if(~isempty(bpth))
      | set_param(char(bpth),'Name',sprintf('%s\n%s','Scissor','Load'),'LinkStatus','none','FontWeight','bold');
      | end
      mask Display: disp('Scissor')
  Use Simple Load : Subsystem
      settings: OpenFcn=|
      | load_system('Cylinder_Lib');
      | load_system('Motor_Lib');
      | load_system('Valve_Lib');
      | load_system('Load_Lib');
      | 
      | bpth = replace_block(bdroot,'Name',sprintf('%s\n%s','Scissor','Load'),'Load_Lib/Simple','noprompt');
      | if(~isempty(bpth))
      | set_param(char(bpth),'Name',sprintf('%s\n%s','Simple','Load'),'LinkStatus','none');               end
      mask Display: disp('Simple')
  Use Standard Actuator : Subsystem
      settings: OpenFcn=|
      | load_system('Cylinder_Lib');
      | load_system('Motor_Lib');
      | load_system('Valve_Lib');
      | load_system('Load_Lib');
      | 
      | bpth = replace_block(bdroot,'Name',sprintf('%s\n%s','Custom','Actuator'),'Cylinder_Lib/Standard','noprompt');
      | if(~isempty(bpth))
      | set_param(char(bpth),'Name',sprintf('%s\n%s','Standard','Actuator'),'LinkStatus','none','FontWeight','bold');
      | end
      mask Display: disp('Standard')
  Use Standard Motor : Subsystem
      settings: OpenFcn=|
      | load_system('Cylinder_Lib');
      | load_system('Motor_Lib');
      | load_system('Valve_Lib');
      | load_system('Load_Lib');
      | 
      | bpth = replace_block(bdroot,'Name',sprintf('%s\n%s','Custom','Servo & Controller'),'Motor_Lib/Standard','noprompt');
      | if(~isempty(bpth))
      | set_param(char(bpth),'Name',sprintf('%s\n%s','Standard','Servo & Controller'),'LinkStatus','none','FontWeight','bold');
      | end
      mask Display: disp('Standard')
  Use Standard Valve : Subsystem
      settings: OpenFcn=|
      | load_system('Cylinder_Lib');
      | load_system('Motor_Lib');
      | load_system('Valve_Lib');
      | load_system('Load_Lib');
      | 
      | bpth = replace_block(bdroot,'Name',sprintf('%s\n%s','Custom','Valve'),'Valve_Lib/Standard','noprompt');
      | if(~isempty(bpth))
      | set_param(char(bpth),'Name',sprintf('%s\n%s','Standard','Valve'),'LinkStatus','none','FontWeight','bold');
      | end
      mask Display: disp('Standard')

== system Hydraulic_Lift/Custom Actuator/Sensing ==
  bar1 : nesl_utility/PS-Simulink Converter  PhysicalDomain=network_engine_domain  SubClassName=ps_output  LeftPortType=input  RightPortType=output  PseudoPeriodic=off  Frequencies=[]  Unit=mm  AffineConversion=off
  S : PMIOPort  Port=1  Side=Left
  tag scope: Disp_Meas=global
  wires:
  bar1/1 -> [Disp_Meas]
  connections:
  bar1/LConn1 -- S/RConn1

== system Hydraulic_Lift/Custom Actuator/Sensor 1 ==
  Hydraulic Reference1 : fl_lib/Hydraulic/Hydraulic Elements/Hydraulic Reference  q_Log=off  LocalVarNames=|q  LocalVarDescs=|q  LocalVarLogging=[]
  Ideal Hydraulic Pressure Sensor : fl_lib/Hydraulic/Hydraulic Sensors/Hydraulic Pressure Sensor  q_Log=off  p_Log=off  LocalVarNames=|q|p  LocalVarDescs=|q|p  LocalVarLogging=[]
  bar1 : nesl_utility/PS-Simulink Converter  PhysicalDomain=network_engine_domain  SubClassName=ps_output  LeftPortType=input  RightPortType=output  PseudoPeriodic=off  Frequencies=[]  Unit=bar  AffineConversion=off
  P : PMIOPort  Port=1  Side=Left
  tag scope: PA=global
  wires:
  bar1/1 -> [PA]
  connections:
  Ideal Hydraulic Pressure Sensor/RConn1 -- Hydraulic Reference1/LConn1
  Ideal Hydraulic Pressure Sensor/RConn2 -- bar1/LConn1
  P/RConn1 -- Ideal Hydraulic Pressure Sensor/LConn1

== system Hydraulic_Lift/Custom Actuator/Sensor 2 ==
  Hydraulic Reference1 : fl_lib/Hydraulic/Hydraulic Elements/Hydraulic Reference  q_Log=off  LocalVarNames=|q  LocalVarDescs=|q  LocalVarLogging=[]
  Ideal Hydraulic Pressure Sensor : fl_lib/Hydraulic/Hydraulic Sensors/Hydraulic Pressure Sensor  q_Log=off  p_Log=off  LocalVarNames=|q|p  LocalVarDescs=|q|p  LocalVarLogging=[]
  bar1 : nesl_utility/PS-Simulink Converter  PhysicalDomain=network_engine_domain  SubClassName=ps_output  LeftPortType=input  RightPortType=output  PseudoPeriodic=off  Frequencies=[]  Unit=bar  AffineConversion=off
  P : PMIOPort  Port=1  Side=Left
  tag scope: PB=global
  wires:
  bar1/1 -> [PB]
  connections:
  P/RConn1 -- Ideal Hydraulic Pressure Sensor/LConn1
  Ideal Hydraulic Pressure Sensor/RConn2 -- bar1/LConn1
  Ideal Hydraulic Pressure Sensor/RConn1 -- Hydraulic Reference1/LConn1

== system Hydraulic_Lift/Custom Servo & Controller/LVDT Position Sensor System 10V//mm ==
  10V/mm : fl_lib/Physical Signals/Functions/PS Gain  gain=10*1000  LocalVarLogging=[]
  Controlled Voltage Source : fl_lib/Electrical/Electrical Sources/Controlled Voltage Source  i_Log=off  v_Log=off  LocalVarNames=|current|voltage|power  LocalVarDescs=|Current (A)|Voltage (V)|Power (W)  LocalVarLogging=[0 0 0]
  Motion Sensor : fl_lib/Mechanical/Mechanical Sensors/Ideal Translational Motion Sensor  offset=0 m  v_Log=off  f_Log=off  x_Log=off  LocalVarNames=|v|f|x  LocalVarDescs=|v|f|x  LocalVarLogging=[0 0 0]
  - : PMIOPort  Port=1  Side=Right
  + : PMIOPort  Port=2  Side=Right
  C : PMIOPort  Port=3  Side=Left
  R : PMIOPort  Port=4  Side=Left
  connections:
  +/RConn1 -- Controlled Voltage Source/LConn1
  -/RConn1 -- Controlled Voltage Source/RConn2
  R/RConn1 -- Motion Sensor/LConn1
  10V/mm/RConn1 -- Controlled Voltage Source/RConn1
  C/RConn1 -- Motion Sensor/RConn1
  Motion Sensor/RConn3 -- 10V/mm/LConn1

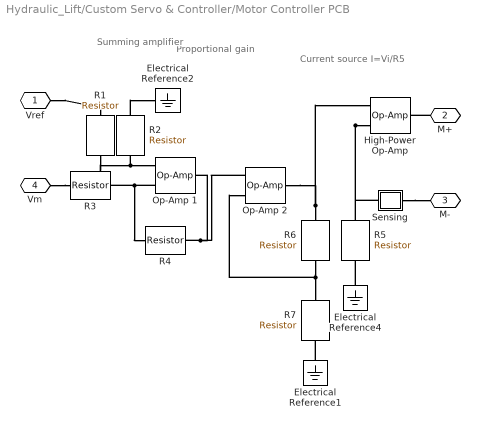
== system Hydraulic_Lift/Custom Servo & Controller/Motor Controller PCB ==
  note: Proportional gain
  note: Summing
      | amplifier
  note: Current source
      | I=Vi/R5
  Electrical Reference1 : fl_lib/Electrical/Electrical Elements/Electrical Reference  i_Log=off  LocalVarNames=|i  LocalVarDescs=|i  LocalVarLogging=[]
  Electrical Reference2 : fl_lib/Electrical/Electrical Elements/Electrical Reference  i_Log=off  LocalVarNames=|i  LocalVarDescs=|i  LocalVarLogging=[]
  Electrical Reference4 : fl_lib/Electrical/Electrical Elements/Electrical Reference  i_Log=off  LocalVarNames=|i  LocalVarDescs=|i  LocalVarLogging=[]
  High-Power Op-Amp : fl_lib/Electrical/Electrical Elements/Op-Amp  i1_Log=off  v1_Log=off  outI_Log=off  LocalVarNames=|i1|v1|outI  LocalVarDescs=|i1|v1|outI  LocalVarLogging=[]
  Op-Amp 1 : fl_lib/Electrical/Electrical Elements/Op-Amp  i1_Log=off  v1_Log=off  outI_Log=off  LocalVarNames=|i1|v1|outI  LocalVarDescs=|i1|v1|outI  LocalVarLogging=[]
  Op-Amp 2 : fl_lib/Electrical/Electrical Elements/Op-Amp  i1_Log=off  v1_Log=off  outI_Log=off  LocalVarNames=|i1|v1|outI  LocalVarDescs=|i1|v1|outI  LocalVarLogging=[]
  R1 : fl_lib/Electrical/Electrical Elements/Resistor  R=R_controller(1) Ohm  i_Log=off  v_Log=off  LocalVarNames=|current|voltage|power  LocalVarDescs=|Resistor current (A)|Voltage across resistor (V)|Power (W)  LocalVarLogging=[0 0 0]
  R2 : fl_lib/Electrical/Electrical Elements/Resistor  R=R_controller(2) Ohm  i_Log=off  v_Log=off  LocalVarNames=|current|voltage|power  LocalVarDescs=|Resistor current (A)|Voltage across resistor (V)|Power (W)  LocalVarLogging=[0 0 0]
  R3 : fl_lib/Electrical/Electrical Elements/Resistor  R=R_controller(3) Ohm  i_Log=off  v_Log=off  LocalVarNames=|current|voltage|power  LocalVarDescs=|Resistor current (A)|Voltage across resistor (V)|Power (W)  LocalVarLogging=[0 0 0]
  R4 : fl_lib/Electrical/Electrical Elements/Resistor  R=R_controller(4) Ohm  i_Log=off  v_Log=off  LocalVarNames=|current|voltage|power  LocalVarDescs=|Resistor current (A)|Voltage across resistor (V)|Power (W)  LocalVarLogging=[0 0 0]
  R5 : fl_lib/Electrical/Electrical Elements/Resistor  R=R_controller(5) Ohm  i_Log=off  v_Log=off  LocalVarNames=|current|voltage|power  LocalVarDescs=|Resistor current (A)|Voltage across resistor (V)|Power (W)  LocalVarLogging=[0 0 0]
  R6 : fl_lib/Electrical/Electrical Elements/Resistor  R=R_controller(6) Ohm  i_Log=off  v_Log=off  LocalVarNames=|current|voltage|power  LocalVarDescs=|Resistor current (A)|Voltage across resistor (V)|Power (W)  LocalVarLogging=[0 0 0]
  R7 : fl_lib/Electrical/Electrical Elements/Resistor  R=R_controller(7) Ohm  i_Log=off  v_Log=off  LocalVarNames=|current|voltage|power  LocalVarDescs=|Resistor current (A)|Voltage across resistor (V)|Power (W)  LocalVarLogging=[0 0 0]
  Sensing : Subsystem
      mask Display: disp('S')
  Vref : PMIOPort  Port=1  Side=Left
  M+ : PMIOPort  Port=2  Side=Right
  M- : PMIOPort  Port=3  Side=Right
  Vm : PMIOPort  Port=4  Side=Left
  connections:
  Sensing/RConn1 -- M-/RConn1
  Vm/RConn1 -- R3/LConn1
  M+/RConn1 -- High-Power Op-Amp/RConn1
  Vref/RConn1 -- R1/LConn1
  R6/RConn1 -- R7/LConn1 -- Op-Amp 2/LConn2
  R4/RConn1 -- Op-Amp 1/RConn1 -- Op-Amp 2/LConn1
  Op-Amp 1/LConn2 -- R4/LConn1 -- R3/RConn1
  R1/RConn1 -- Op-Amp 1/LConn1 -- R2/LConn1
  High-Power Op-Amp/LConn2 -- Sensing/LConn1 -- R5/LConn1
  R6/LConn1 -- Op-Amp 2/RConn1 -- High-Power Op-Amp/LConn1
  Electrical Reference4/LConn1 -- R5/RConn1
  R2/RConn1 -- Electrical Reference2/LConn1
  Electrical Reference1/LConn1 -- R7/RConn1

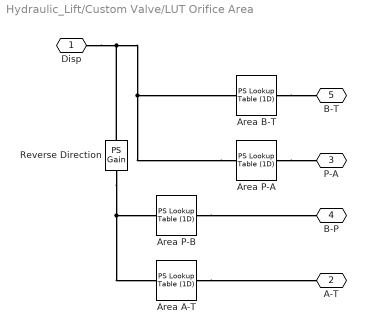
== system Hydraulic_Lift/Custom Valve/LUT Orifice Area ==
  Area A-T : fl_lib/Physical Signals/Lookup Tables/PS Lookup Table (1D)  x_t=[-x_max -x_lap 0 x_lap x_max 2*x_max]*1e-3  y_t=[0 0 A_leak 2*A_leak A_max A_max]*1e-6  interp_method=1  extrap_method=1  LocalVarLogging=[]
  Area B-T : fl_lib/Physical Signals/Lookup Tables/PS Lookup Table (1D)  x_t=[-x_max -x_lap 0 x_lap x_max 2*x_max]*1e-3  y_t=[0 0 A_leak 2*A_leak A_max A_max]*1e-6  interp_method=1  extrap_method=1  LocalVarLogging=[]
  Area P-A : fl_lib/Physical Signals/Lookup Tables/PS Lookup Table (1D)  x_t=[-x_max -x_lap 0 x_lap x_max 2*x_max]*1e-3  y_t=[0 0 A_leak 2*A_leak A_max A_max]*1e-6  interp_method=1  extrap_method=1  LocalVarLogging=[]
  Area P-B : fl_lib/Physical Signals/Lookup Tables/PS Lookup Table (1D)  x_t=[-x_max -x_lap 0 x_lap x_max 2*x_max]*1e-3  y_t=[0 0 A_leak 2*A_leak A_max A_max]*1e-6  interp_method=1  extrap_method=1  LocalVarLogging=[]
  Reverse Direction : fl_lib/Physical Signals/Functions/PS Gain  gain=-1  LocalVarLogging=[]
  Disp : PMIOPort  Port=1  Side=Left
  A-T : PMIOPort  Port=2  Side=Right
  P-A : PMIOPort  Port=3  Side=Right
  B-P : PMIOPort  Port=4  Side=Right
  B-T : PMIOPort  Port=5  Side=Right
  connections:
  Area P-A/RConn1 -- P-A/RConn1
  Area P-A/LConn1 -- Area B-T/LConn1 -- Reverse Direction/LConn1 -- Disp/RConn1
  Area B-T/RConn1 -- B-T/RConn1
  Reverse Direction/RConn1 -- Area P-B/LConn1 -- Area A-T/LConn1
  Area P-B/RConn1 -- B-P/RConn1
  Area A-T/RConn1 -- A-T/RConn1

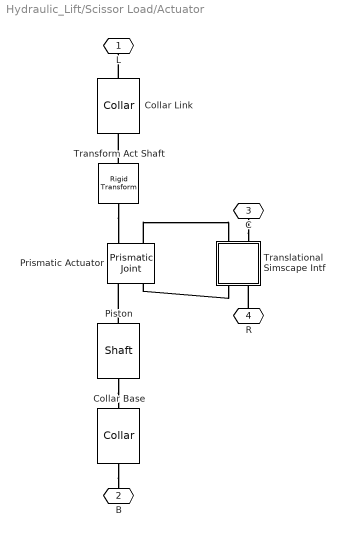
== system Hydraulic_Lift/Scissor Load/Actuator ==
  Collar Base : Scissor_Parts_Lib/Collar  collar_length=Scissor_Lift_Param.Actuator.Collar.Length  collar_radius=Scissor_Lift_Param.Actuator.Collar.Radius  cylinder_length=Scissor_Lift_Param.Actuator.Piston_Seat.Length*2  cylinder_radius=Scissor_Lift_Param.Actuator.Piston_Seat.Radius  cylinder_ori=Local +Z  material_density=Scissor_Lift_Param.Actuator.Collar.Density  material_color=Scissor_Lift_Param.Actuator.Collar.Color  material_opacity=Scissor_Lift_Param.Actuator.Collar.Opacity
  Collar Link : Scissor_Parts_Lib/Collar  collar_length=Scissor_Lift_Param.Actuator.Collar.Length  collar_radius=Scissor_Lift_Param.Actuator.Collar.Radius  cylinder_length=Scissor_Lift_Param.Actuator.Piston_Seat.Length*2  cylinder_radius=Scissor_Lift_Param.Actuator.Piston_Seat.Radius  cylinder_ori=Local +Z  material_density=Scissor_Lift_Param.Actuator.Collar.Density  material_color=Scissor_Lift_Param.Actuator.Collar.Color  material_opacity=Scissor_Lift_Param.Actuator.Collar.Opacity
  Piston : Scissor_Parts_Lib/Shaft  L=Scissor_Lift_Param.Actuator.Piston.Length  r=Scissor_Lift_Param.Actuator.Piston.Radius  theta=0  z_ori=Local +Z  Ro=Scissor_Lift_Param.Actuator.Piston.Density  clr=Scissor_Lift_Param.Actuator.Piston.Color  opc=Scissor_Lift_Param.Actuator.Piston.Opacity
  Prismatic Actuator : sm_lib/Joints/Prismatic  Joint  SenseConstraintForceX=off  SenseConstraintForceY=off  SenseConstraintForceZ=off  SenseConstraintTorqueX=off  SenseConstraintTorqueY=off  SenseConstraintTorqueZ=off  ConstraintWrenchDir=FollowerOnBase  ConstraintWrenchFrame=BaseFrame  EquilibriumPosition=0  EquilibriumPositionUnits=m  SpringStiffness=0  SpringStiffnessUnits=N/m  DampingCoefficient=Scissor_Lift_Param.Actuator.Damping  DampingCoefficientUnits=N/(m/s)  ActuationMode=TorqueForceActuation  SensePosition=off  SenseVelocity=on  SenseAcceleration=off  SenseTorqueForce=off  PositionTargetValue=0  PositionTargetValueUnits=m  PositionTargetSpecify=off  PositionTargetPriority=High  VelocityTargetValue=0  VelocityTargetValueUnits=m/s  VelocityTargetSpecify=off  VelocityTargetPriority=High  BlockFunction=simmechanics.library.joints.prismatic_joint
  Transform Act Shaft : sm_lib/Frames and  Transforms/Rigid  Transform  TranslationMethod=None  TranslationLengthUnit=cm  TranslationStandardAxis=-X  TranslationStandardOffset=0  TranslationCartesianOffset=[0 0 0]  TranslationROffset=0  TranslationROffsetUnits=m  TranslationZOffset=0  TranslationZOffsetUnits=m  TranslationThetaOffset=0  TranslationThetaOffsetUnits=deg  RotationMethod=StandardAxis  RotationAngleUnits=deg  RotationStandardAxis=+X  RotationAngle=180  RotationArbitraryAxis=[0 0 1]  FollAlignAxisA=+X  BaseAlignAxisA=+Y  FollAlignAxisB=+Y  BaseAlignAxisB=+Z  BlockFunction=simmechanics.library.frames_transforms.rigid_transform
  Translational Simscape Intf : Subsystem
  L : PMIOPort  Port=1  Side=Right
  B : PMIOPort  Port=2  Side=Left
  C : PMIOPort  Port=3  Side=Left
  R : PMIOPort  Port=4  Side=Right
  connections:
  Collar Base/LConn1 -- B/RConn1
  Transform Act Shaft/RConn1 -- Prismatic Actuator/LConn1
  Prismatic Actuator/LConn2 -- Translational Simscape Intf/LConn1
  Translational Simscape Intf/RConn1 -- Prismatic Actuator/RConn2
  Collar Link/LConn1 -- L/RConn1
  Transform Act Shaft/LConn1 -- Collar Link/RConn1
  Piston/LConn1 -- Collar Base/RConn1
  Piston/RConn1 -- Prismatic Actuator/RConn1
  C/RConn1 -- Translational Simscape Intf/LConn2
  R/RConn1 -- Translational Simscape Intf/RConn2
